simulink model "Modelo_panel"  (R2025a)
settings: Solver=VariableStepAuto  StartTime=0.0  StopTime=10.0  RelTol=1e-3
undefined symbols (not defined in the file): Iscref, Np, Ns, Voc
libraries: SignalEditorBlockLib x1
settings Model: Creator=Rodri  LastModifiedBy=BSLAY

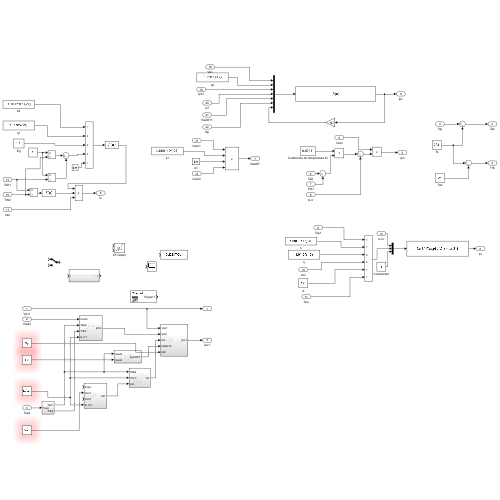
[thumbnail: Simulink's stored preview of the top-level diagram]
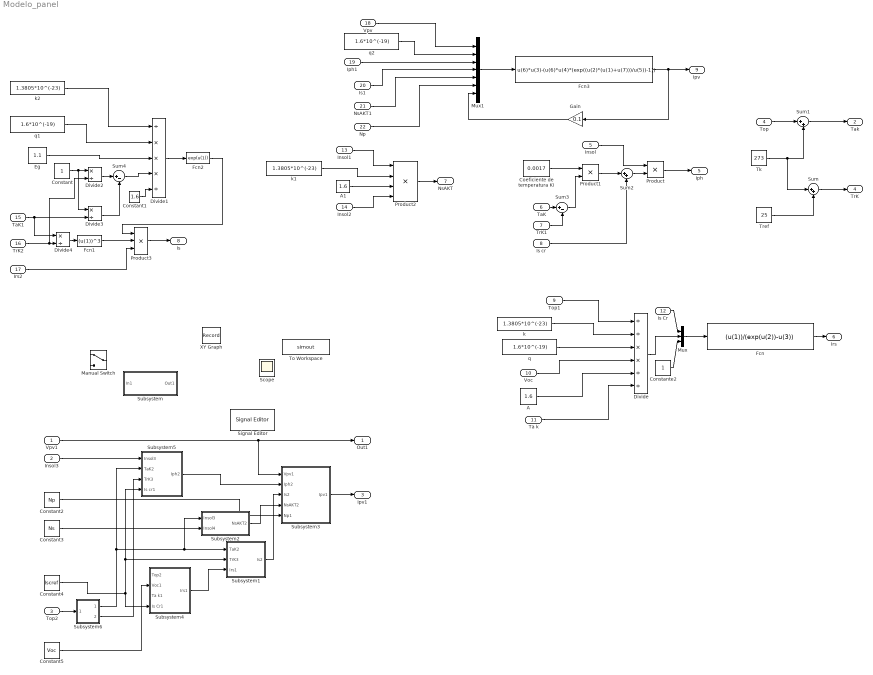
== system Modelo_panel ==
  Vpv1 : Inport
  Insol3 : Inport  Port=2
  Top2 : Inport  Port=3
  Top : Inport  Port=4
  Insol : Inport  Port=5
  TaK : Inport  Port=6
  TrK1 : Inport  Port=7
  Is cr : Inport  Port=8
  Top1 : Inport  Port=9
  Voc : Inport  Port=10
  Ta k : Inport  Port=11
  Is Cr : Inport  Port=12
  Insol1 : Inport  Port=13
  Insol2 : Inport  Port=14
  TaK1 : Inport  Port=15
  TrK2 : Inport  Port=16
  Irs2 : Inport  Port=17
  Vpv : Inport  Port=18
  Iph1 : Inport  Port=19
  Is1 : Inport  Port=20
  NsAKT1 : Inport  Port=21
  Np : Inport  Port=22
  A : Constant  Value=1.6
  A1 : Constant  Value=1.6
  Coeficiente de temperatura Ki : Constant  Value=0.0017
  Constant : Constant
  Constant1 : Constant  Value=1.6
  Constant2 : Constant  Value=Np
  Constant3 : Constant  Value=Ns
  Constant4 : Constant  Value=Iscref
  Constant5 : Constant  Value=Voc
  Constante2 : Constant
  Divide : Product  Inputs=//**//
  Divide1 : Product  Inputs=/***/
  Divide2 : Product  Inputs=*/
  Divide3 : Product  Inputs=*/
  Divide4 : Product  Inputs=*/
  Eg : Constant  Value=1.1
  Fcn : Fcn  Expr=(u(1))/(exp(u(2))-u(3))
  Fcn1 : Fcn  Expr=(u(1))^3
  Fcn2 : Fcn  Expr=exp(u(1))
  Fcn3 : Fcn  Expr=u(6)*u(3)-(u(6)*u(4)*(exp((u(2)*(u(1)+u(7)))/u(5))-1))
  Gain : Gain  Gain=0.1
  Manual Switch : ManualSwitch
  Mux : Mux  Inputs=3
  Mux1 : Mux  Inputs=7
  Product : Product
  Product1 : Product
  Product2 : Product  Inputs=4
  Product3 : Product  Inputs=3
  Scope : Scope
  Signal Editor : SignalEditorBlockLib/Signal Editor  FileName=untitled.mat  ActiveScenario=Scenario  ActiveSignal=Signal 1  IsBus=off  OutputBusObjectStr=Bus: BusObject  SampleTime=0  Interpolate=off  ZeroCross=off  OutputAfterFinalValue=Setting to zero  Unit=inherit  PreserveSignalName=on  ApplySigPropsToAllScenarios=on  ApplySigPropsToAllSignals=off  SignalPropertySource=Dialog parameters
  Subsystem : Subsystem
  Subsystem1 : Subsystem
  Subsystem2 : Subsystem
  Subsystem3 : Subsystem
  Subsystem4 : Subsystem
  Subsystem5 : Subsystem
  Subsystem6 : Subsystem
  Sum : Sum  Inputs=|++
  Sum1 : Sum  Inputs=|++
  Sum2 : Sum  Inputs=|++
  Sum3 : Sum  Inputs=|+-
  Sum4 : Sum  Inputs=|+-
  Tk : Constant  Value=273
  To Workspace : ToWorkspace  VariableName=simout  SaveFormat=Timeseries  SampleTime=-1
  Tref : Constant  Value=25
  XY Graph : Record  NumPorts=2.0  FileSettingsInternal="{\"entries\":[{\"content\":{\"excelSettings\":{\"content\":{},\"type\":\"Streamout.ExcelSettings\"},\"parquetSettings\":{\"content\":{},\"type\":\"Streamout.ParquetSettings\"}},\"type\":\"Streamout.FileSettingStorage\",\"uuid\":\"\"}],\"packageUris\":[\"http:\\/\\/schema.mathworks.com\\/mf0\\/streamout_blocks\\/R2020a\"],\"version\":\"1.0\"}"  FrameSettings=[0, 0]  Layout=[1 1]  SignalsInternal="{\"entries\":[{\"content\":{\"signals\":[{\"content\":{\"blockPath\":[],\"dimensions\":[1],\"domain\":\"\",\"lineColor\":\"#a2142f\",\"plots\":[ 1 ],\"port\":1,\"signalID\":1,\"signalName\":\"XY Graph:1\"},\"type\":\"RecordBlkView.Signal\",\"uuid\":\"\"},{\"content\":{\"blockPath\":[],\"dimensions\":[1],\"domain\":\"\",\"lineColor\":\"#139fff\",\"plots\":[ 1 ],\"port\":2,\"signalID\":2,\"signalName\":\"XY Graph:2\"},\"type\":\"RecordBlkView.Signal\",\"uuid\":\"\"}]},\"type\":\"RecordBlkView.InputSignals\",\"uuid\":\"\"}],\"packageUris\":[\"http:\\/\\/schema.mathworks.com\\/mf0\\/streamout_blocks\\/R2020a\"],\"version\":\"1.0\"}"  VisualizationBindings="{\"xyplotplugin\":{\"info\":[{\"series\":[{\"bindingParametersList\":[{\"parameter\":\"X-Axis\",\"signalID\":1,\"signalName\":\"XY Graph:1\"},{\"parameter\":\"Y-Axis\",\"signalID\":2,\"signalName\":\"XY Graph:2\"}],\"seriesID\":0}],\"subplotID\":1}]}}"  CompatibilityTag=XY
  k : Constant  Value=1.3805*10^(-23)
  k1 : Constant  Value=1.3805*10^(-23)
  k2 : Constant  Value=1.3805*10^(-23)
  q : Constant  Value=1.6*10^(-19)
  q1 : Constant  Value=1.6*10^(-19)
  q2 : Constant  Value=1.6*10^(-19)
  Out1 : Outport
  Tak : Outport  Port=2
  Ipv1 : Outport  Port=3
  TrK : Outport  Port=4
  Iph : Outport  Port=5
  Irs : Outport  Port=6
  NsAKT : Outport  Port=7
  Is : Outport  Port=8
  Ipv : Outport  Port=9
  wires:
  Top/1 -> Sum1/1
  Sum1/1 -> Tak/1
  Tk/1 -> Sum/1, Sum1/2
  Tref/1 -> Sum/2
  Sum/1 -> TrK/1
  Product/1 -> Iph/1
  Coeficiente de temperatura Ki/1 -> Product1/1
  Sum3/1 -> Product1/2
  Product1/1 -> Sum2/1
  Sum2/1 -> Product/2
  Insol/1 -> Product/1
  TaK/1 -> Sum3/1
  TrK1/1 -> Sum3/2
  Is cr/1 -> Sum2/2
  Top1/1 -> Divide/1
  Divide/1 -> Mux/2
  Mux/1 -> Fcn/1
  Fcn/1 -> Irs/1
  k/1 -> Divide/2
  q/1 -> Divide/3
  A/1 -> Divide/5
  Voc/1 -> Divide/4
  Ta k/1 -> Divide/6
  Is Cr/1 -> Mux/1
  Constante2/1 -> Mux/3
  Insol2/1 -> Product2/4
  Insol1/1 -> Product2/1
  Product2/1 -> NsAKT/1
  A1/1 -> Product2/3
  k1/1 -> Product2/2
  k2/1 -> Divide1/1
  q1/1 -> Divide1/2
  Divide2/1 -> Sum4/1
  Eg/1 -> Divide1/3
  Constant/1 -> Divide3/1, Divide2/1
  Sum4/1 -> Divide1/4
  TaK1/1 -> Divide4/1, Divide3/2
  TrK2/1 -> Divide2/2, Divide4/2
  Irs2/1 -> Product3/3
  Divide4/1 -> Fcn1/1
  Fcn1/1 -> Product3/2
  Divide1/1 -> Fcn2/1
  Fcn2/1 -> Product3/1
  Divide3/1 -> Sum4/2
  Constant1/1 -> Divide1/5
  Product3/1 -> Is/1
  Gain/1 -> Mux1/7
  Fcn3/1 -> Gain/1, Ipv/1
  Mux1/1 -> Fcn3/1
  Vpv/1 -> Mux1/1
  q2/1 -> Mux1/2
  Iph1/1 -> Mux1/3
  Np/1 -> Mux1/6
  NsAKT1/1 -> Mux1/5
  Is1/1 -> Mux1/4
  Vpv1/1 -> Subsystem3/1(Vpv1), Out1/1
  Subsystem3/1(Ipv1) -> Ipv1/1
  Insol3/1 -> Subsystem5/1(Insol3)
  Subsystem5/1(Iph2) -> Subsystem3/2(Iph2)
  Top2/1 -> Subsystem6/1(Top2)
  Subsystem6/1(Tak1) -> Subsystem5/2(TaK2), Subsystem2/1(Insol3), Subsystem1/1(TaK2)
  Subsystem6/2(TrK3) -> Subsystem5/3(TrK3)
  Subsystem2/1(NsAKT2) -> Subsystem3/4(NsAKT2)
  Constant2/1 -> Subsystem3/5(Np1)
  Subsystem1/1(Is2) -> Subsystem3/3(Is2)
  Constant3/1 -> Subsystem2/2(Insol4)
  Constant5/1 -> Subsystem4/2(Voc1)
  Constant4/1 -> Subsystem5/4(Is cr1), Subsystem1/2(TrK3), Subsystem4/4(Is Cr1)
  Subsystem4/1(Irs1) -> Subsystem1/3(Irs1)

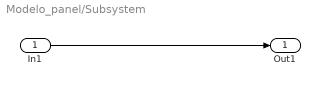
== system Modelo_panel/Subsystem ==
  In1 : Inport
  Out1 : Outport
  wires:
  In1/1 -> Out1/1

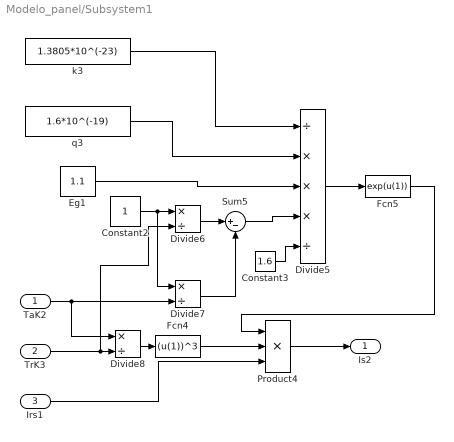
== system Modelo_panel/Subsystem1 ==
  TaK2 : Inport
  TrK3 : Inport  Port=2
  Irs1 : Inport  Port=3
  Constant2 : Constant
  Constant3 : Constant  Value=1.6
  Divide5 : Product  Inputs=/***/
  Divide6 : Product  Inputs=*/
  Divide7 : Product  Inputs=*/
  Divide8 : Product  Inputs=*/
  Eg1 : Constant  Value=1.1
  Fcn4 : Fcn  Expr=(u(1))^3
  Fcn5 : Fcn  Expr=exp(u(1))
  Product4 : Product  Inputs=3
  Sum5 : Sum  Inputs=|+-
  k3 : Constant  Value=1.3805*10^(-23)
  q3 : Constant  Value=1.6*10^(-19)
  Is2 : Outport
  wires:
  Divide5/1 -> Fcn5/1
  TaK2/1 -> Divide8/1, Divide7/2
  k3/1 -> Divide5/1
  Irs1/1 -> Product4/3
  Constant3/1 -> Divide5/5
  Fcn5/1 -> Product4/1
  Product4/1 -> Is2/1
  TrK3/1 -> Divide6/2, Divide8/2
  Eg1/1 -> Divide5/3
  Constant2/1 -> Divide7/1, Divide6/1
  Divide6/1 -> Sum5/1
  Divide7/1 -> Sum5/2
  q3/1 -> Divide5/2
  Fcn4/1 -> Product4/2
  Divide8/1 -> Fcn4/1
  Sum5/1 -> Divide5/4

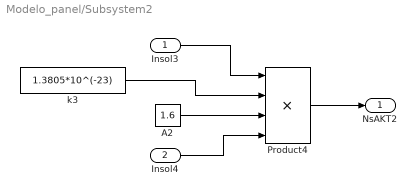
== system Modelo_panel/Subsystem2 ==
  Insol3 : Inport
  Insol4 : Inport  Port=2
  A2 : Constant  Value=1.6
  Product4 : Product  Inputs=4
  k3 : Constant  Value=1.3805*10^(-23)
  NsAKT2 : Outport
  wires:
  Insol3/1 -> Product4/1
  Product4/1 -> NsAKT2/1
  k3/1 -> Product4/2
  A2/1 -> Product4/3
  Insol4/1 -> Product4/4

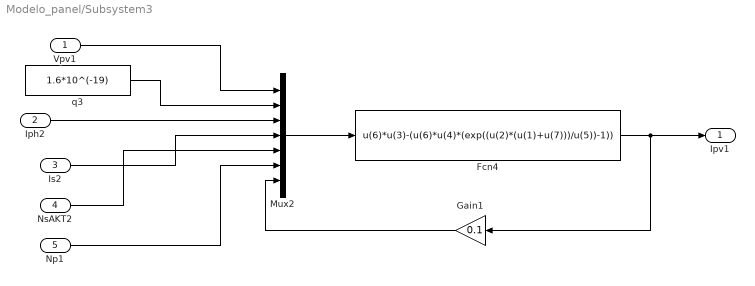
== system Modelo_panel/Subsystem3 ==
  Vpv1 : Inport
  Iph2 : Inport  Port=2
  Is2 : Inport  Port=3
  NsAKT2 : Inport  Port=4
  Np1 : Inport  Port=5
  Fcn4 : Fcn  Expr=u(6)*u(3)-(u(6)*u(4)*(exp((u(2)*(u(1)+u(7)))/u(5))-1))
  Gain1 : Gain  Gain=0.1
  Mux2 : Mux  Inputs=7
  q3 : Constant  Value=1.6*10^(-19)
  Ipv1 : Outport
  wires:
  q3/1 -> Mux2/2
  Is2/1 -> Mux2/4
  Mux2/1 -> Fcn4/1
  Gain1/1 -> Mux2/7
  NsAKT2/1 -> Mux2/5
  Iph2/1 -> Mux2/3
  Fcn4/1 -> Ipv1/1, Gain1/1
  Vpv1/1 -> Mux2/1
  Np1/1 -> Mux2/6

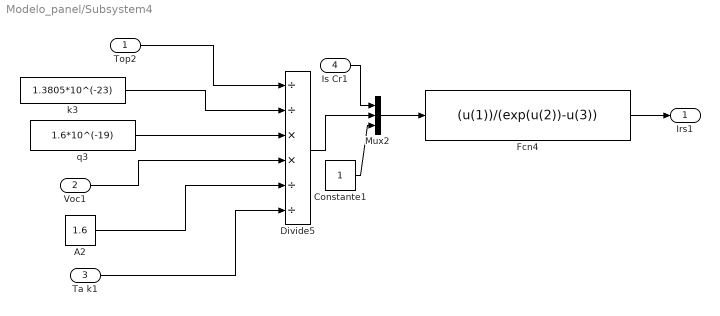
== system Modelo_panel/Subsystem4 ==
  Top2 : Inport
  Voc1 : Inport  Port=2
  Ta k1 : Inport  Port=3
  Is Cr1 : Inport  Port=4
  A2 : Constant  Value=1.6
  Constante1 : Constant
  Divide5 : Product  Inputs=//**//
  Fcn4 : Fcn  Expr=(u(1))/(exp(u(2))-u(3))
  Mux2 : Mux  Inputs=3
  k3 : Constant  Value=1.3805*10^(-23)
  q3 : Constant  Value=1.6*10^(-19)
  Irs1 : Outport
  wires:
  Fcn4/1 -> Irs1/1
  A2/1 -> Divide5/5
  Ta k1/1 -> Divide5/6
  Top2/1 -> Divide5/1
  Divide5/1 -> Mux2/2
  q3/1 -> Divide5/3
  Constante1/1 -> Mux2/3
  k3/1 -> Divide5/2
  Voc1/1 -> Divide5/4
  Mux2/1 -> Fcn4/1
  Is Cr1/1 -> Mux2/1

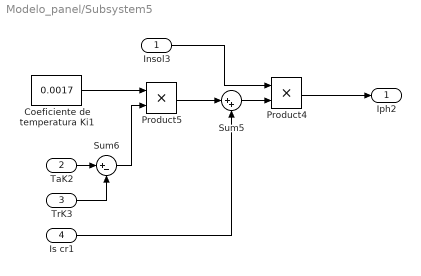
== system Modelo_panel/Subsystem5 ==
  Insol3 : Inport
  TaK2 : Inport  Port=2
  TrK3 : Inport  Port=3
  Is cr1 : Inport  Port=4
  Coeficiente de temperatura Ki1 : Constant  Value=0.0017
  Product4 : Product
  Product5 : Product
  Sum5 : Sum  Inputs=|++
  Sum6 : Sum  Inputs=|+-
  Iph2 : Outport
  wires:
  Product5/1 -> Sum5/1
  Sum6/1 -> Product5/2
  Sum5/1 -> Product4/2
  TaK2/1 -> Sum6/1
  Product4/1 -> Iph2/1
  Is cr1/1 -> Sum5/2
  TrK3/1 -> Sum6/2
  Coeficiente de temperatura Ki1/1 -> Product5/1
  Insol3/1 -> Product4/1

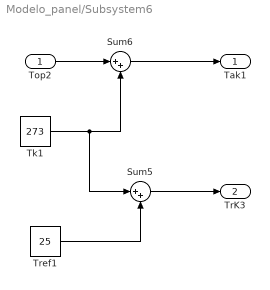
== system Modelo_panel/Subsystem6 ==
  Top2 : Inport
  Sum5 : Sum  Inputs=|++
  Sum6 : Sum  Inputs=|++
  Tk1 : Constant  Value=273
  Tref1 : Constant  Value=25
  Tak1 : Outport
  TrK3 : Outport  Port=2
  wires:
  Sum6/1 -> Tak1/1
  Top2/1 -> Sum6/1
  Tref1/1 -> Sum5/2
  Tk1/1 -> Sum5/1, Sum6/2
  Sum5/1 -> TrK3/1
